simulink model "cessna_doublet"  (R2026a)
settings: Solver=ode45  StopTime=tfinal  MaxStep=.001
values from neighbouring files (symbols this model uses):
  UStar = temp.UStar    [sim_doublet_cessna.m]    (also in trim_30ms.mat = [-0.120172368527 0.107844993241]; trim_40ms.mat = [-0.0341598178801 0.170728091655]; trim_50ms.mat = [0.00593898652725 0.261948782149]; trim_60ms.mat = [0.0277937749516 0.386870836155])
  XStar = temp.XStar    [sim_doublet_cessna.m]    (also in trim_30ms.mat = [28.7880822315 8.44075360558 -4.45531014099e-13 0.2852094575; trim_40ms.mat = [39.6739046846 5.09718423039 -4.21568544513e-13 0.1277770239; trim_50ms.mat = [49.9260818807 2.71778366307 -9.92968512818e-13 0.0543824749; trim_60ms.mat = [59.9937959493 0.862813767865 3.22570290237e-12 0.0143807251)
undefined symbols (not defined in the file or in its folder): cessna182_model, degtorad
settings Model: Creator=nuris  LastModifiedBy=nuris

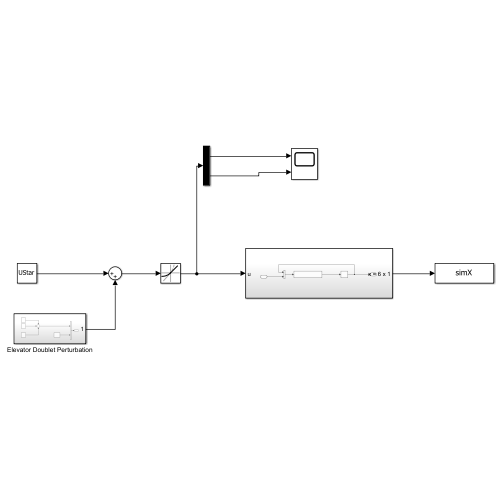
[thumbnail: Simulink's stored preview of the top-level diagram]
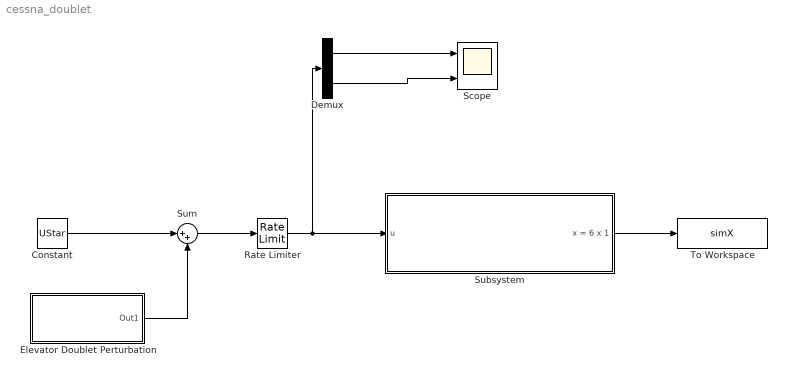
== system cessna_doublet ==
  Constant : Constant  Value=UStar
  Demux : Demux  Outputs=2
  Elevator Doublet Perturbation : Subsystem
  Rate Limiter : RateLimiter  RisingSlewLimit=deg2rad(5)  FallingSlewLimit=-deg2rad(10)  SampleTimeMode=inherited
  Scope : Scope  NumInputPorts=2
      settings: ActiveDisplayYMinimum=-0.045141886695815509  ActiveDisplayYMaximum=0.12106180450333376
  Subsystem : Subsystem
  Sum : Sum  Inputs=|++
  To Workspace : ToWorkspace  VariableName=simX  SaveFormat=Timeseries  SampleTime=-1
  wires:
  Subsystem/1(x = 6 x 1) -> To Workspace/1
  Demux/1 -> Scope/1
  Demux/2 -> Scope/2
  Constant/1 -> Sum/1
  Elevator Doublet Perturbation/1(Out1) -> Sum/2
  Sum/1 -> Rate Limiter/1
  Rate Limiter/1 -> Demux/1, Subsystem/1(u)

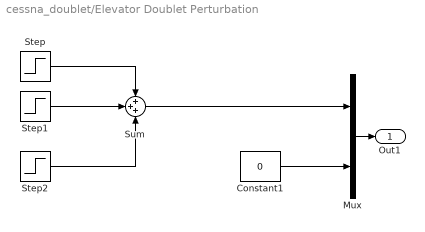
== system cessna_doublet/Elevator Doublet Perturbation ==
  Constant1 : Constant  Value=0
  Mux : Mux  Inputs=2
  Step : Step  FinalValue=degtorad(5)  SampleTime=0
  Step1 : Step  Time=5  FinalValue=-degtorad(10)  SampleTime=0
  Step2 : Step  Time=9  FinalValue=degtorad(5)  SampleTime=0
  Sum : Sum  Inputs=+++
  Out1 : Outport
  wires:
  Step1/1 -> Sum/2
  Mux/1 -> Out1/1
  Step/1 -> Sum/1
  Constant1/1 -> Mux/2
  Sum/1 -> Mux/1
  Step2/1 -> Sum/3

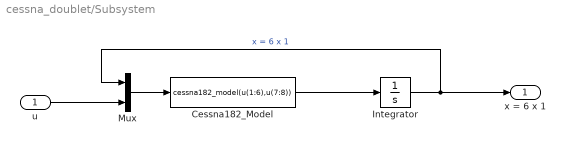
== system cessna_doublet/Subsystem ==
  u : Inport
  Cessna182_Model : MATLABFcn  MATLABFcn=cessna182_model(u(1:6),u(7:8))
  Integrator : Integrator  InitialCondition=XStar
  Mux : Mux  Inputs=2
  x = 6 x 1 : Outport
  wires:
  Cessna182_Model/1 -> Integrator/1
  Integrator/1 -> Mux/1, x = 6 x 1/1  "x = 6 x 1"
  Mux/1 -> Cessna182_Model/1
  u/1 -> Mux/2
